simulink model "huamo4ws"  (R2024b)
settings: Solver=VariableStepAuto  StartTime=0.0  StopTime=10  RelTol=1e-3
values from neighbouring files (symbols this model uses):
  A = [(Kf+Kr)/m/v (a*Kf-Kr)/m/v/v-1;(a*Kf-b*Kr)/Iz (a*a*Kf+b*b*Kr)/Iz/v]    [canshu.m]
  B = [-Kf/m/v;-a*Kf/Iz]    [canshu.m]
libraries: Solver_SF x1
settings Model: Creator=28677  LastModifiedBy=28677

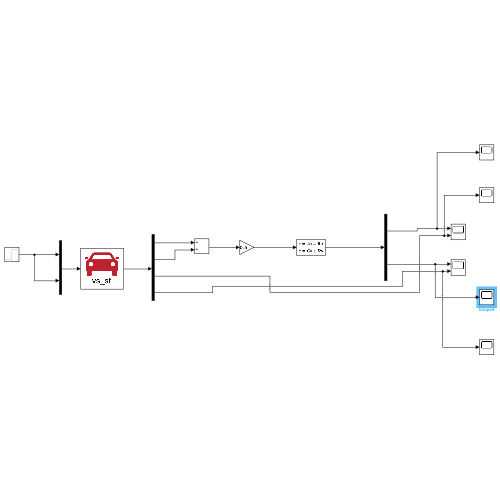
[thumbnail: Simulink's stored preview of the top-level diagram]
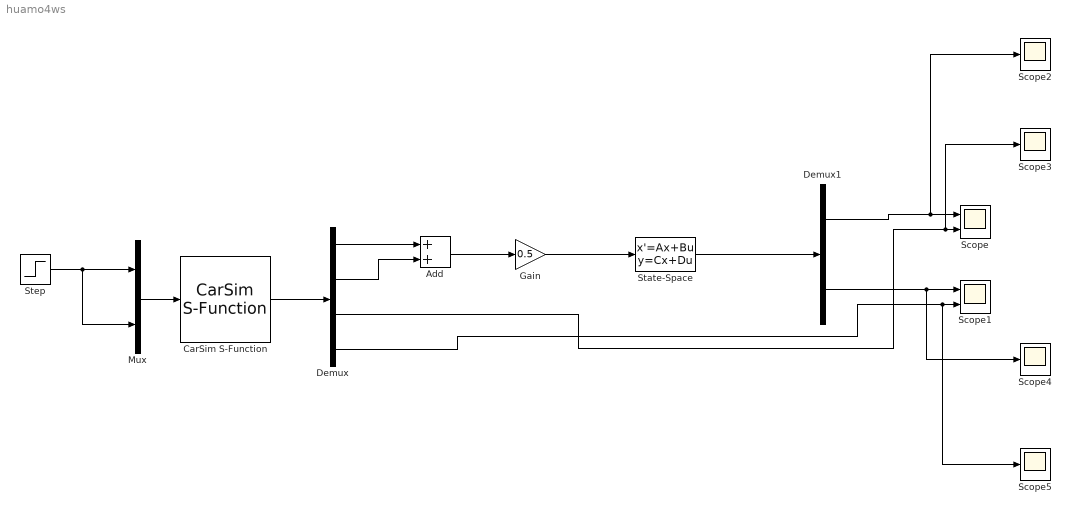
== system huamo4ws ==
  Add : Sum
  CarSim S-Function : Solver_SF/CarSim S-Function  Priority=1  SIMFILE=simfile.sim  Run_RTs=off  vs_state_ind=Run  StopMode_ind=Vehicle Model
  Demux : Demux
  Demux1 : Demux  Outputs=2
  Gain : Gain  Gain=0.5
  Mux : Mux  Inputs=2
  Scope : Scope  NumInputPorts=2
  Scope1 : Scope  NumInputPorts=2
  Scope{2..5} (4 alike) : Scope
  State-Space : StateSpace  A=A  B=B  C=eye(2)  D=zeros(2,1)  InitialCondition=0
  Step : Step  SampleTime=0
  wires:
  Mux/1 -> CarSim S-Function/1
  Step/1 -> Mux/2, Mux/1
  CarSim S-Function/1 -> Demux/1
  Demux/1 -> Add/1
  Demux/2 -> Add/2
  Add/1 -> Gain/1
  Demux1/1 -> Scope2/1, Scope/1
  Demux1/2 -> Scope4/1, Scope1/1
  Demux/3 -> Scope3/1, Scope/2
  Demux/4 -> Scope5/1, Scope1/2
  Gain/1 -> State-Space/1
  State-Space/1 -> Demux1/1
